simulink model "sevietta_devel_2017h"  (R2013a)
settings: Solver=VariableStepDiscrete  SolverMode=SingleTasking  StartTime=0.0  StopTime=3276  RelTol=1e-3
undefined symbols (not defined in the file): sfp
libraries: xbsIndex_r4 x2565, casper_library_delays x32, simulink x19, casper_library_misc x17, xps_library x13
(part 1 of 31)
settings Model: Creator=jkocz  LastModifiedBy=dancpr
settings Model: ModifiedComment=|
  | dancpr -- Tue May 02 13:59:12 2017 -- Version 1.666
  | 
  | Changed down to 48 dead time cycles between packets. Also fixed bram name issue.
settings Model: ModifiedHistory=|
  | dancpr -- Tue May 02 13:59:12 2017 -- Version 1.666
  | 
  | Changed down to 48 dead time cycles between packets. Also fixed bram name issue.
  | 
  | dancpr -- Tue May 02 11:03:32 2017 -- Version 1.665
  | 
  | Changed dead time from 64 --> 128
  | 
  | dancpr -- Tue May 02 10:58:43 2017 -- Version 1.664
  | 
  | Changing dead time between EOF and SOF to improve max line rate for LWA-SV 6 subbands
  | 
  | dancpr -- Wed Apr 26 22:03:29 2017 -- Version 1.663
  | 
  | 
  | dancpr -- Wed Apr 26 21:41:13 2017 -- Version 1.662
  | 
  | 
  | dancpr -- Wed Apr 26 16:23:23 2017 -- Version 1.661
  | 
  | 
  | dancpr -- Wed Apr 26 14:02:39 2017 -- Version 1.660
  | Added gbe3 - see if it compiles...
  | 
  | dancpr -- Wed Apr 26 13:58:47 2017 -- Version 1.659
  | 
  | 
  | dancpr -- Wed Apr 26 13:54:04 2017 -- Version 1.658
  | 
  | 
  | dancpr -- Wed Apr 26 10:09:47 2017 -- Version 1.657
  | 
  | 
  | dancpr -- Tue Apr 25 15:28:37 2017 -- Version 1.656
  | 
  | changed start_stop logic to be 14 bits
  | 
  | dancpr -- Tue Apr 25 12:47:41 2017 -- Version 1.655
  | 
  | Changed to 10 GbE on port 3
  | 
  | dancpr -- Tue Apr 25 09:30:05 2017 -- Version 1.654
  | 
  | 
  | dancpr -- Tue Apr 25 09:29:16 2017 -- Version 1.653
  | 
  | 
  | dancpr -- Tue Apr 25 09:23:27 2017 -- Version 1.652
  | 
  | Adding 1gbe port
  | 
  | dancpr -- Wed Mar 08 19:03:55 2017 -- Version 1.651
  | 
  | 
  | dancpr -- Fri Feb 17 15:33:23 2017 -- Version 1.650
  | 
  | Changing start/stop chan to reconfigure without adc_rst
  | 
  | dancpr -- Wed Feb 15 09:42:04 2017 -- Version 1.649
  | 
  | Flipping antenna remap @ cram stage
  | 
  | dancpr -- Tue Feb 14 13:51:39 2017 -- Version 1.648
  | 
  | 
  | dancpr -- Mon Feb 13 23:39:57 2017 -- Version 1.647
  | 
  | weird remap to match jayces request...
  | 
  | dancpr -- Mon Feb 13 12:23:26 2017 -- Version 1.646
  | Added in antenna remap block. Might need to look in to why this remap is happening, it is in blocks of 8 which is hard to understand where this is coming in.
  | 
  | dancpr -- Mon Feb 13 12:23:10 2017 -- Version 1.645
  | 
  | 
  | dancpr -- Thu Feb 09 10:54:23 2017 -- Version 1.644
  | 
  | 
  | dancpr -- Thu Feb 09 10:29:28 2017 -- Version 1.643
  | 
  | 
  | dancpr -- Thu Feb 09 10:21:04 2017 -- Version 1.642
  | 
  | Changed re_logic to be reset by adc_rst -> sync_rnd goto
  | 
  | dancpr -- Wed Feb 08 17:56:33 2017 -- Version 1.641
  | 
  | Now using SOW to reset pkt logic
  | 
  | dancpr -- Wed Feb 08 17:55:55 2017 -- Version 1.640
  | 
  | 
  | dancpr -- Wed Feb 08 17:48:51 2017 -- Version 1.639
  | 
  | 
  | dancpr -- Wed Feb 08 14:38:54 2017 -- Version 1.638
  | 
  | 
  | dancpr -- Wed Feb 08 14:38:18 2017 -- Version 1.637
  | 
  | Changed fifo_en port on packetizer to only go high on sync_rnd, but it will then stay high
  | 
  | dancpr -- Wed Feb 08 14:28:38 2017 -- Version 1.636
  | 
  | 
  | dancpr -- Wed Feb 08 14:18:16 2017 -- Version 1.635
  | 
  | updated all registers to be triggered off sync_rnd reset instead of fft_window. Also found that coarse delay slices were wrong bits :/. Fixed in this version.
  | 
  | dancpr -- Wed Feb 08 14:17:58 2017 -- Version 1.634
  | 
  | 
  | dancpr -- Wed Feb 08 09:19:10 2017 -- Version 1.633
  | 
  | 
  | dancpr -- Wed Feb 08 09:18:22 2017 -- Version 1.632
  | 
  | 
  | dancpr -- Tue Feb 07 21:28:18 2017 -- Version 1.631
  | 
  | 
  | dancpr -- Tue Feb 07 18:42:13 2017 -- Version 1.630
  | 
  | 
  | dancpr -- Tue Feb 07 18:19:40 2017 -- Version 1.629
  | 
  | 
  | dancpr -- Tue Feb 07 14:28:19 2017 -- Version 1.628
  | 
  | 
  | dancpr -- Tue Feb 07 14:24:49 2017 -- Version 1.627
  | 
  | 
  | dancpr -- Tue Feb 07 08:20:11 2017 -- Version 1.626
  | 
  | 
  | dancpr -- Mon Feb 06 13:28:37 2017 -- Version 1.625
  | 
  | 
  | dancpr -- Mon Feb 06 13:25:53 2017 -- Version 1.624
  | 
  | 
  | dancpr -- Mon Feb 06 13:24:37 2017 -- Version 1.623
  | 
  | 
  | dancpr -- Mon Feb 06 13:23:20 2017 -- Version 1.622
  | 
  | simplified packetizer logic
  | 
  | dancpr -- Mon Feb 06 13:09:16 2017 -- Version 1.621
  | 
  | 
  | dancpr -- Mon Feb 06 13:07:33 2017 -- Version 1.620
  | 
  | Changed reset logic for updating registers
  | 
  | dancpr -- Mon Feb 06 10:41:23 2017 -- Version 1.619
  | 
  | 
  | dancpr -- Thu Feb 02 11:13:10 2017 -- Version 1.618
  | 
  | 
  | dancpr -- Thu Feb 02 10:54:04 2017 -- Version 1.617
  | 
  | 
  | dancpr -- Wed Feb 01 23:19:27 2017 -- Version 1.616
  | 
  | 
  | dancpr -- Wed Feb 01 23:18:25 2017 -- Version 1.615
  | 
  | Added 64 bit counter for testing sync logic
  | 
  | dancpr -- Tue Jan 31 18:52:06 2017 -- Version 1.614
  | 
  | 
  | dancpr -- Tue Jan 31 18:49:34 2017 -- Version 1.613
  | 
  | fixed stupid coarse delay bug (bad wiring)
  | 
  | dancpr -- Tue Jan 31 18:40:22 2017 -- Version 1.612
  | 
  | 
  | dancpr -- Tue Jan 31 18:05:38 2017 -- Version 1.611
  | 
  | Increased size of packet buffer from 1024 -> 4096. This allows up to 1024 channels total to be sent via 10 gbe
  | 
  | dancpr -- Tue Jan 31 18:05:02 2017 -- Version 1.610
  | 
  | 
  | dancpr -- Tue Jan 31 18:03:01 2017 -- Version 1.609
  | 
  | 
  | dancpr -- Tue Jan 31 16:59:21 2017 -- Version 1.608
  | 
  | 
  | dancpr -- Tue Jan 31 16:55:53 2017 -- Version 1.607
  | 
  | now have per antpol coarse delay of up to 1024 cycles
  | 
  | dancpr -- Tue Jan 31 13:34:00 2017 -- Version 1.606
  | 
  | 
  | dancpr -- Tue Jan 31 13:33:41 2017 -- Version 1.605
  | 
  | 
  | dancpr -- Tue Jan 31 10:15:03 2017 -- Version 1.604
  | 
  | 
  | dancpr -- Tue Jan 31 10:07:29 2017 -- Version 1.603
  | 
  | 
  | dancpr -- Tue Jan 31 10:05:35 2017 -- Version 1.602
  | 
  | 
  | dancpr -- Wed Dec 21 01:24:07 2016 -- Version 1.601
  | 
  | 
  | dancpr -- Wed Dec 21 01:23:19 2016 -- Version 1.600
  | 
  | Changed the offset in f-engine from 5 to 2
  | 
  | dancpr -- Tue Dec 20 20:26:40 2016 -- Version 1.599
  | 
  | 
  | dancpr -- Sun Dec 18 17:08:23 2016 -- Version 1.598
  | 
  | 
  | dancpr -- Sun Dec 18 17:03:59 2016 -- Version 1.597
  | 
  | 
  | dancpr -- Fri Dec 16 02:52:14 2016 -- Version 1.596
  | 
  | Changed sync logic
  | 
  | dancpr -- Thu Dec 15 20:01:21 2016 -- Version 1.595
  | 
  | 
  | dancpr -- Thu Dec 15 13:10:24 2016 -- Version 1.594
  | 
  | Added in test vector into design, selectable by mux
  | 
  | dancpr -- Thu Dec 15 13:09:58 2016 -- Version 1.593
  | 
  | 
  | dancpr -- Wed Dec 14 16:25:37 2016 -- Version 1.592
  | 
  | 
  | dancpr -- Wed Dec 14 16:23:09 2016 -- Version 1.591
  | 
  | stopped rst_seq_num resetting FIFO
  | 
  | dancpr -- Tue Dec 06 23:15:00 2016 -- Version 1.590
  | 
  | 
  | dancpr -- Mon Dec 05 15:37:36 2016 -- Version 1.589
  | 
  | 
  | dancpr -- Mon Dec 05 15:33:46 2016 -- Version 1.588
  | 
  | 
  | dancpr -- Sun Dec 04 15:08:55 2016 -- Version 1.587
  | 
  | Adding in delay offset as mentioned by Jayce
  | 
  | dancpr -- Sat Dec 03 10:16:37 2016 -- Version 1.586
  | 
  | 
  | dancpr -- Sat Dec 03 07:16:08 2016 -- Version 1.585
  | 
  | 
  | dancpr -- Sat Dec 03 07:13:03 2016 -- Version 1.584
  | 
  | 
  | dancpr -- Sat Dec 03 01:12:31 2016 -- Version 1.583
  | 
  | 
  | dancpr -- Sat Dec 03 01:11:28 2016 -- Version 1.582
  | 
  | 
  | dancpr -- Sat Dec 03 01:06:45 2016 -- Version 1.581
  | 
  | 
  | dancpr -- Sat Dec 03 01:05:35 2016 -- Version 1.580
  | 
  | Added coarse delay in, max 2^10 cycle delay
  | 
  | dancpr -- Sat Dec 03 00:33:46 2016 -- Version 1.579
  | 
  | 
  | dancpr -- Fri Dec 02 16:14:28 2016 -- Version 1.578
  | 
  | 
  | dancpr -- Fri Dec 02 16:13:55 2016 -- Version 1.577
  | 
  | 
  | dancpr -- Fri Dec 02 14:58:19 2016 -- Version 1.576
  | 
  | 
  | dancpr -- Fri Dec 02 14:56:26 2016 -- Version 1.575
  | added fifo_en back in
  | 
  | dancpr -- Thu Dec 01 23:33:25 2016 -- Version 1.574
  | 
  | 
  | dancpr -- Thu Dec 01 23:29:07 2016 -- Version 1.573
  | 
  | 
  | dancpr -- Thu Dec 01 23:25:09 2016 -- Version 1.572
  | 
  | 
  | dancpr -- Thu Dec 01 16:39:14 2016 -- Version 1.571
  | 
  | 
  | dancpr -- Thu Dec 01 15:20:38 2016 -- Version 1.570
  | 
  | 
  | dancpr -- Thu Dec 01 15:18:56 2016 -- Version 1.569
  | 
  | 
  | dancpr -- Thu Dec 01 13:44:08 2016 -- Version 1.568
  | 
  | 
  | dancpr -- Thu Dec 01 09:16:00 2016 -- Version 1.567
  | 
  | 
  | dancpr -- Wed Nov 30 23:48:09 2016 -- Version 1.566
  | 
  | 
  | dancpr -- Wed Nov 30 16:14:18 2016 -- Version 1.565
  | 
  | 
  | dancpr -- Wed Nov 30 14:18:38 2016 -- Version 1.564
  | adding in random delay on EOF
  | 
  | dancpr -- Wed Nov 30 12:47:12 2016 -- Version 1.563
  | 
  | 
  | dancpr -- Wed Nov 30 12:44:03 2016 -- Version 1.562
  | 
  | 
  | dancpr -- Wed Nov 30 12:41:48 2016 -- Version 1.561
  | 
  | 
  | dancpr -- Wed Nov 30 12:40:58 2016 -- Version 1.560
  | 
  | 
  | dancpr -- Wed Nov 30 12:36:33 2016 -- Version 1.559
  | 
  | 
  | dancpr -- Wed Nov 30 12:36:04 2016 -- Version 1.558
  | 
  | 
  | dancpr -- Wed Nov 30 12:28:10 2016 -- Version 1.557
  | 
  | 
  | dancpr -- Wed Nov 30 12:12:31 2016 -- Version 1.556
  | 
  | Major rehaul of register update
  | 
  | dancpr -- Wed Nov 30 11:00:37 2016 -- Version 1.555
  | 
  | 
  | dancpr -- Wed Nov 30 10:22:41 2016 -- Version 1.554
  | 
  | 
  | dancpr -- Wed Nov 30 10:02:31 2016 -- Version 1.553
  | 
  | 
  | dancpr -- Wed Nov 30 09:54:42 2016 -- Version 1.552
  | 
  | 
  | dancpr -- Wed Nov 30 09:47:40 2016 -- Version 1.551
  | 
  | 
  | dancpr -- Wed Nov 30 09:26:22 2016 -- Version 1.550
  | 
  | 
  | dancpr -- Wed Nov 30 00:29:05 2016 -- Version 1.549
  | 
  | 
  | dancpr -- Wed Nov 30 00:08:37 2016 -- Version 1.548
  | 
  | 
  | dancpr -- Wed Nov 30 00:00:00 2016 -- Version 1.547
  | 
  | 
  | dancpr -- Tue Nov 29 23:48:50 2016 -- Version 1.546
  | 
  | 
  | dancpr -- Tue Nov 29 23:35:12 2016 -- Version 1.545
  | 
  | 
  | dancpr -- Tue Nov 29 23:05:07 2016 -- Version 1.544
  | 
  | 
  | dancpr -- Tue Nov 29 22:42:17 2016 -- Version 1.543
  | 
  | 
  | dancpr -- Tue Nov 29 16:14:41 2016 -- Version 1.542
  | 
  | 
  | dancpr -- Sun Nov 27 23:05:16 2016 -- Version 1.541
  | 
  | Changed counter thingo to be 64 bit
  | 
  | dancpr -- Sun Nov 27 20:43:14 2016 -- Version 1.540
  | 
  | 
  | dancpr -- Sun Nov 27 20:42:36 2016 -- Version 1.539
  | 
  | 
  | dancpr -- Sat Nov 26 15:29:43 2016 -- Version 1.538
  | 
  | 
  | dancpr -- Sat Nov 26 15:09:52 2016 -- Version 1.537
  | 
  | 
  | dancpr -- Wed Nov 23 14:58:51 2016 -- Version 1.536
  | 
  | WILL TRY A COMPILE IN STYLE
  | 
  | dancpr -- Wed Nov 23 14:36:45 2016 -- Version 1.535
  | 
  | 
  | dancpr -- Wed Nov 23 14:36:16 2016 -- Version 1.534
  | 
  | 
  | dancpr -- Thu Nov 03 16:40:11 2016 -- Version 1.533
  | 
  | 
  | dancpr -- Thu Nov 03 14:30:02 2016 -- Version 1.532
  | 
  | 
  | dancpr -- Thu Nov 03 14:17:22 2016 -- Version 1.531
  | 
  | 
  | dancpr -- Thu Nov 03 14:08:17 2016 -- Version 1.530
  | 
  | 
  | dancpr -- Thu Nov 03 12:20:22 2016 -- Version 1.529
  | 
  | 
  | dancpr -- Thu Nov 03 12:06:52 2016 -- Version 1.528
  | 
  | 
  | dancpr -- Sun Oct 30 20:07:53 2016 -- Version 1.527
  | 
  | 
  | dancpr -- Sun Oct 30 20:05:41 2016 -- Version 1.526
  | 
  | Informed by Jack that the gbe core does not like to be reset. Moved reset logic for the core to a dedicated register
  | 
  | dancpr -- Fri Oct 21 15:11:54 2016 -- Version 1.525
  | 
  | 
  | dancpr -- Fri Oct 21 15:10:49 2016 -- Version 1.524
  | 
  | 
  | dancpr -- Thu Oct 20 13:55:11 2016 -- Version 1.523
  | 
  | 
  | dprice -- Thu Sep 29 17:00:09 2016 -- Version 1.522
  | 
  | 10GbE core now resets when tx_enable goes high
  | 
  | dprice -- Wed Sep 28 20:28:10 2016 -- Version 1.521
  | 
  | Added sync through fft_bypass mux, combined changes from version 2016g firmware.
  | 
  | dprice -- Wed Sep 28 20:19:32 2016 -- Version 1.520
  | 
  | 
  | dprice -- Wed Sep 14 19:32:07 2016 -- Version 1.519
  | 
  | 
  | dprice -- Wed Sep 14 15:23:18 2016 -- Version 1.518
  | 
  | 
  | dprice -- Wed Sep 14 15:16:21 2016 -- Version 1.517
  | 
  | Hardcoding stuff
  | 
  | dprice -- Wed Mar 30 11:54:00 2016 -- Version 1.516
  | 
  | Removed VACC to try and meet timing!
  | 
  | dprice -- Tue Mar 29 21:49:47 2016 -- Version 1.515
  | 
  | Changed vacc DSP48E for vacc simple
  | 
  | dprice -- Tue Mar 29 12:17:53 2016 -- Version 1.514
  | Remove coarse delay to help meet timing :/
  | 
  | dprice -- Tue Mar 29 12:08:09 2016 -- Version 1.513
  | 
  | 
  | dprice -- Mon Mar 28 16:01:17 2016 -- Version 1.512
  | added pipeline delays in vacc to help timing
  | 
  | dprice -- Fri Mar 25 15:35:21 2016 -- Version 1.511
  | 
  | 
  | dprice -- Fri Mar 25 15:28:38 2016 -- Version 1.510
  | 
  | 
  | dprice -- Fri Mar 25 15:12:44 2016 -- Version 1.509
  | 
  | 
  | dprice -- Fri Mar 25 15:01:55 2016 -- Version 1.508
  | 
  | 
  | dprice -- Fri Mar 25 15:00:46 2016 -- Version 1.507
  | 
  | 
  | dprice -- Fri Mar 25 14:47:25 2016 -- Version 1.506
  | 
  | 
  | dprice -- Fri Mar 25 14:33:41 2016 -- Version 1.505
  | 
  | 
  | dprice -- Fri Mar 25 14:32:44 2016 -- Version 1.504
  | Updated blocks to casper_astro_devel
  | 
  | dprice -- Fri Mar 25 14:01:45 2016 -- Version 1.503
  | 
  | 
  | dprice -- Fri Mar 25 13:10:40 2016 -- Version 1.502
  | 
  | Updated coarse delay and added extra pipelining on vacc
  | 
  | dprice -- Fri Mar 25 12:55:40 2016 -- Version 1.501
  | 
  | 
  | dprice -- Mon Mar 21 15:41:15 2016 -- Version 1.500
  | 
  | 
  | dprice -- Fri Mar 18 16:50:06 2016 -- Version 1.499
  | 
  | Added n_roach software register, at Ben's request
  | 
  | dprice -- Fri Mar 18 12:55:02 2016 -- Version 1.498
  | 
  | 
  | dprice -- Wed Mar 16 17:10:07 2016 -- Version 1.497
  | 
  | 
  | dprice -- Wed Mar 16 16:18:52 2016 -- Version 1.496
  | 
  | added in FFT bypass
  | 
  | dprice -- Wed Mar 16 15:57:40 2016 -- Version 1.495
  | 
  | 
  | dprice -- Fri Feb 12 17:29:32 2016 -- Version 1.494
  | 
  | 
  | dprice -- Fri Feb 12 17:17:53 2016 -- Version 1.493
  | 
  | 
  | dprice -- Fri Feb 12 16:48:45 2016 -- Version 1.492
  | 
  | Using leda512_2016e, with updated FFT and spectrometer, with sevietta_devel3 packetizer
  | 
  | dprice -- Fri Feb 12 16:42:59 2016 -- Version 1.491
  | 
  | 
  | dprice -- Mon Feb 01 14:04:02 2016 -- Version 1.490
  | 
  | Added pipeline delays after eq blocks
  | 
  | dprice -- Fri Jan 29 13:04:51 2016 -- Version 1.489
  | 
  | Added pipeline delays on pfb_fir as the timing logs showed this as an issue
  | 
  | dprice -- Wed Jan 27 14:02:19 2016 -- Version 1.488
  | 
  | Changed FFT core
  | 
  | dprice -- Wed Jan 27 13:22:12 2016 -- Version 1.487
  | 
  | Using latest casper_astro_devel more recent FFT
  | 
  | dprice -- Fri Jan 22 10:59:16 2016 -- Version 1.486
  | Added in old tenge core
  | 
  | dprice -- Fri Jan 22 10:26:56 2016 -- Version 1.485
  | about to change tengbe block out
  | 
  | dprice -- Thu Jan 21 17:16:55 2016 -- Version 1.484
  | 
  | 
  | dprice -- Wed Jan 20 11:44:21 2016 -- Version 1.483
  | 
  | Added pipelines around requant mux to help timing
  | 
  | dprice -- Tue Jan 19 16:58:53 2016 -- Version 1.482
  | 
  | 
  | dprice -- Tue Jan 19 16:57:42 2016 -- Version 1.481
  | 
  | added in coarse delay after ADC
  | 
  | dprice -- Tue Jan 19 16:48:56 2016 -- Version 1.480
  | 
  | 
  | dprice -- Tue Jan 19 16:38:05 2016 -- Version 1.479
  | 
  | 
  | dprice -- Tue Jan 19 16:27:23 2016 -- Version 1.478
  | Adding coarse delay
  | 
  | dprice -- Tue Jan 19 15:47:20 2016 -- Version 1.477
  | 
  | 
  | dprice -- Tue Jan 19 15:44:29 2016 -- Version 1.476
  | 
  | 
  | dprice -- Thu Jan 07 01:25:30 2016 -- Version 1.475
  | 
  | Removed goddam FFT preshift shift
  | 
  | dprice -- Mon Jan 04 15:23:51 2016 -- Version 1.474
  | 
  | changed acc_cnt to run up to 2^25 = 1 year
  | 
  | dprice -- Mon Dec 28 14:47:04 2015 -- Version 1.473
  | 
  | Changed requant mux yet again, now can choose in 2 bit steps, from LSB up to -4 from MSB. This will clip RFI
  | 
  | dprice -- Tue Dec 22 18:17:34 2015 -- Version 1.472
  | 
  | Now using simplest requant imaginable: 18 bit slice. Changed vacc toa accept 18 bits, output 32 bits. Allows 14 bits of growth = 2^14 cycles = 16384 cycles = OK
  | 
  | dprice -- Tue Dec 22 18:10:53 2015 -- Version 1.471
  | 
  | 
  | dprice -- Tue Dec 22 16:37:14 2015 -- Version 1.470
  | 
  | Changed bitsel once again, -4 increments
  | 
  | dprice -- Sat Dec 19 20:03:40 2015 -- Version 1.469
  | 
  | Now slicing tops bits only -- can choose 0 - 4 bit offset (12 dB dynamic range). This is more than the sky changes, so should be OK?
  | 
  | dprice -- Thu Dec 17 17:05:01 2015 -- Version 1.468
  | 
  | Changed spectrometer quantization rq
  | 
  | dprice -- Tue Dec 15 08:55:34 2015 -- Version 1.467
  | 
  | Added pipeline delays in tenge block - may have broken something...
  | 
  | dprice -- Tue Dec 15 00:02:55 2015 -- Version 1.466
  | 
  | added dealys before rq mux to help timing. hopefully it compiles now.
  | 
  | dprice -- Mon Dec 14 21:02:26 2015 -- Version 1.465
  | 
  | adding delays back in to see if timing affected. I probably screwed up EOF by just removing it anyways.
  | 
  | dprice -- Mon Dec 14 21:01:23 2015 -- Version 1.464
  | 
  | adding pipeline delay
  | 
  | dprice -- Mon Dec 14 17:37:49 2015 -- Version 1.463
  | 
  | changed spectrometer requeant to do 18_17 -> 16_15.
  | 
  | Removed some random delays in the tenge to see what happens
  | 
  | dprice -- Mon Dec 14 17:35:29 2015 -- Version 1.462
  | 
  | 
  | dprice -- Tue Dec 08 15:27:01 2015 -- Version 1.461
  | 
  | changed requant to just slice the bits of interest
  | 
  | dprice -- Tue Dec 08 15:08:55 2015 -- Version 1.460
  | 
  | Added fft preshift, and fixed bit offset in rq
  | 
  | dprice -- Mon Apr 06 20:09:48 2015 -- Version 1.459
  | Compiled successfully
  | 
  | dprice -- Mon Apr 06 16:18:15 2015 -- Version 1.458
  | 
  | Changed pps delay to about 0.1s
  | 
  | dprice -- Fri Mar 13 15:46:33 2015 -- Version 1.457
  | 
  | 
  | dprice -- Fri Mar 13 15:34:50 2015 -- Version 1.456
  | Copied triggering over to f1 - f4
  | 
  | dprice -- Fri Mar 13 15:31:03 2015 -- Version 1.455
  | 
  | Added better triggering of RMS monitor
  | 
  | dprice -- Wed Jan 21 17:17:07 2015 -- Version 1.454
  | 
  | 
  | dprice -- Wed Jan 21 14:02:39 2015 -- Version 1.453
  | changed to be triggered by correct pps
  | 
  | dprice -- Thu Jan 15 16:51:06 2015 -- Version 1.452
  | dropped core back to 200 MHz from 216 MHz
  | 
  | dprice -- Thu Jan 15 13:30:59 2015 -- Version 1.451
  | 
  | Changed to use PPS triggered vacc. Needs testing!
  | 
  | dprice -- Thu Jan 15 13:21:59 2015 -- Version 1.450
  | 
  | 
  | dprice -- Thu Jan 15 13:19:39 2015 -- Version 1.449
  | 
  | 
  | dprice -- Thu Jan 15 13:13:52 2015 -- Version 1.448
  | 
  | Adding pps triggered vacc
  | 
  | dprice -- Tue Jan 13 15:35:09 2015 -- Version 1.447
  | 
  | Updated to spectrometer f_engine core
  | 
  | dprice -- Wed Dec 17 17:14:12 2014 -- Version 1.446
  | 
  | added some snap blocks to do eq0 output rms tests
  | 
  | dprice -- Fri Nov 21 18:19:20 2014 -- Version 1.445
  | 
  | 
  | dprice -- Fri Nov 21 15:29:28 2014 -- Version 1.444
  | 
  | 
  | dprice -- Fri Nov 21 15:28:21 2014 -- Version 1.443
  | 
  | 
  | dprice -- Fri Nov 21 15:22:12 2014 -- Version 1.442
  | 
  | About to try a compile
  | 
  | dprice -- Fri Nov 21 15:19:27 2014 -- Version 1.441
  | 
  | 
  | dprice -- Fri Nov 21 15:10:28 2014 -- Version 1.440
  | 
  | about to crash :/
  | 
  | dprice -- Thu Dec 19 14:05:55 2013 -- Version 1.439
  | 
  | Removed scope blocks in 10GbE spacketizer
  | 
  | dprice -- Thu Dec 12 01:39:04 2013 -- Version 1.438
  | 
  | Moved pfb and eq to black boxes. Hopefully compile times are a little quicker now...
  | 
  | dprice -- Wed Dec 11 11:19:03 2013 -- Version 1.437
  | 
  | Updated coeff generator (cg) with separate sky BRAM for switching (sw_sky), renamed sky to bpass, and changed from 18 bit to 32 bit coefficients
  | 
  | dprice -- Tue Dec 10 14:55:05 2013 -- Version 1.436
  | 
  | Closing session
  | 
  | dprice -- Sat Dec 07 16:46:59 2013 -- Version 1.435
  | Fixed bool slicing on tgbe_en
  | 
  | dprice -- Wed Dec 04 22:02:25 2013 -- Version 1.434
  | 
  | Trying to compile with 4x gbes in the design
  | 
  | dprice -- Wed Dec 04 21:44:55 2013 -- Version 1.433
  | 
  | Added extra tgbe blocks for failover
  | 
  | dprice -- Wed Dec 04 17:45:31 2013 -- Version 1.432
  | 
  | Renamed coeff_gen cg to save on length of bram name
  | 
  | dprice -- Wed Dec 04 17:38:25 2013 -- Version 1.431
  | 
  | Copied logic across to all fft/fX blocks. Trying first compile.
  | 
  | dprice -- Wed Dec 04 17:29:39 2013 -- Version 1.430
  | 
  | Modified eq block to allow selecting between switched and all-sky modes
  | 
  | dprice -- Wed Dec 04 16:56:15 2013 -- Version 1.429
  | 
  | Adding switching assembly coefficient selection by pps
  | 
  | dprice -- Wed Nov 06 11:09:49 2013 -- Version 1.428
  | 
  | Changed back down to 216 MHz. Added a post-eq snap block for testing of equalization levels
  | 
  | dprice -- Tue Nov 05 18:21:00 2013 -- Version 1.427
  | 
  | Removed scopes as they bring up an irritating message each time you try and compile
  | 
  | dprice -- Tue Nov 05 14:30:34 2013 -- Version 1.426
  | 
  | Found timing issues with round block. Added a mask and increased latency in convert and multiply.
  | 
  | dprice -- Tue Nov 05 11:43:26 2013 -- Version 1.423
  | 
  | Changed clock to 239 MHz, just to see if it still compiles...
  | 
  | dprice -- Tue Nov 05 11:43:26 2013 -- Version 1.423
  | 
  | Changed clock to 239 MHz, just to see if it still compiles...
  | 
  | dprice -- Tue Nov 05 09:11:40 2013 -- Version 1.422
  | 
  | Design compiled successfully at 210 MHz using pblock constraints (hstack). Now bumping to 216 MHz.
  | Added status LEDs to design for PPS and TX
  | 
  | dprice -- Mon Nov 04 16:36:08 2013 -- Version 1.421
  | 
  | Added pipeline delays to yelllow block I/O in effort to aid timing. Worst offending net was the rst yellow block, presumably due to fanout.
  | 
  | Also modified the ADC thresholding logic to use a BRAM vector accumulator.
  | 
  | dprice -- Tue Oct 29 13:55:56 2013 -- Version 1.412
  | 
  | Fixed mux error - due to goto tag mismatch
  | 
  | dprice -- Tue Oct 29 13:55:56 2013 -- Version 1.412
  | 
  | Fixed mux error - due to goto tag mismatch
  | 
  | dprice -- Tue Oct 29 11:53:04 2013 -- Version 1.411
  | 
  | WTF is wrong with these mux blocks? Keep getting error on dtype in on muxes in packetbuffer.
  | 
  | dprice -- Mon Oct 28 18:12:23 2013 -- Version 1.410
  | 
  | 
  | dprice -- Mon Oct 28 18:11:25 2013 -- Version 1.409
  | 
  | Need to remove slice on FFT_SHIFTS
  | 
  | * Black boxed FFT
  | * Added ADC overflow logic and snap.
settings DataIOCC: SignalLoggingSaveFormat=ModelDataLogs
settings OptimizationCC: InlineParams=on  ExpressionDepthLimit=2147483647
settings DebuggingCC: FcnCallInpInsideContextMsg=UseLocalSettings  StrictBusMsg=Warning
settings GRTTargetCC: CombineOutputUpdateFcns=off  GRTInterface=on

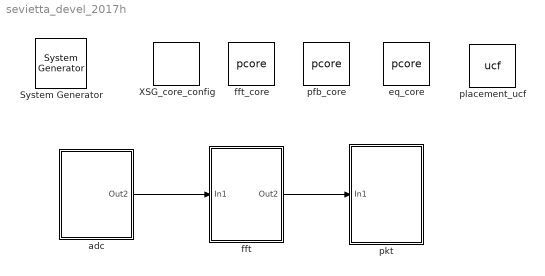
== system sevietta_devel_2017h ==
  " System Generator" : xbsIndex_r4/ System Generator  Tag=genX  xilinxfamily=virtex6  part=xc6vsx475t  speed=-1  package=ff1759  synthesis_tool=XST  clock_wrapper=Clock Enables  directory=./sevietta_devel_2017h/sysgen  proj_type=Project Navigator  Synth_file=XST Defaults  Impl_file=ISE Defaults  testbench=off  simulink_period=1  sysclk_period=4.878  dcm_input_clock_period=100  incr_netlist=off  trim_vbits=Everywhere in SubSystem  dbl_ovrd=According to Block Masks  core_generation=According to Block Masks  run_coregen=off  deprecated_control=off  eval_field=0  block_type=sysgen
      settings: block_version=11.4
  XSG_core_config : xps_library/XSG_core_config  Tag=xps:xsg  hw_sys=ROACH2:sx475t  clk_src=adc0_clk  ROACH_clk_src=sys_clk  ROACH2_clk_src=adc0_clk  MKDIG_clk_src=sys_clk  clk_rate=205  sample_period=1  synthesis_tool=XST
  adc : Subsystem
  eq_core : xps_library/pcore  Tag=xps:pcore  pcore_path=/home/dancpr/leda_firmware/roach_firmware/firmware_2016/bb/cores/eq_basic_core.ngc
  fft : Subsystem
  fft_core : xps_library/pcore  Tag=xps:pcore  pcore_path=/home/dancpr/leda_firmware/roach_firmware/firmware_2016/bb/cores/fft_astro_devel_core.ngc
  pfb_core : xps_library/pcore  Tag=xps:pcore  pcore_path=/home/dancpr/leda_firmware/roach_firmware/firmware_2016/bb/cores/pfb_core.ngc
  pkt : Subsystem
  placement_ucf : xps_library/ucf  Tag=xps:ucf  ucf_file=/home/dancpr/leda_firmware/roach_firmware/placement/l512_fft_quandrants.ucf
  wires:
  adc/1(Out2) -> fft/1(In1)
  fft/1(Out2) -> pkt/1(In1)
